simulink model "simulink_model_undamped"  (R2022b)
settings: Solver=ode5  StartTime=0.0  StopTime=10.0  RelTol=1e-3
settings Model: Creator=Cole  LastModifiedBy=Cole
settings DataIOCC: ReturnWorkspaceOutputs=off

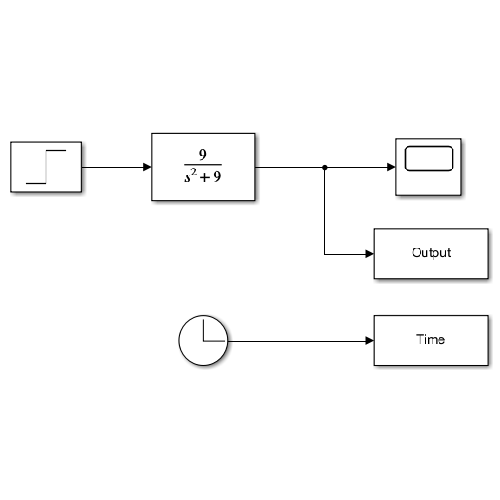
[thumbnail: Simulink's stored preview of the top-level diagram]
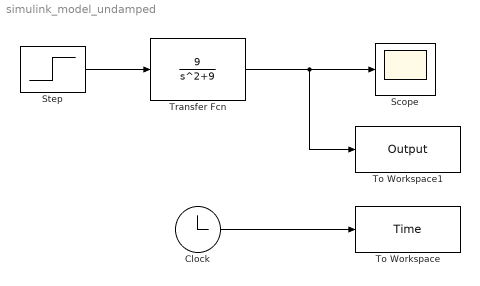
== system simulink_model_undamped ==
  Clock : Clock
  Scope : Scope
  Step : Step  Time=0  SampleTime=0
  To Workspace : ToWorkspace  VariableName=Time  SaveFormat=Timeseries  SampleTime=-1
  To Workspace1 : ToWorkspace  VariableName=Output  SaveFormat=Timeseries  SampleTime=-1
  Transfer Fcn : TransferFcn  Numerator=[9]  Denominator=[1 0 9]
  wires:
  Step/1 -> Transfer Fcn/1
  Transfer Fcn/1 -> Scope/1, To Workspace1/1
  Clock/1 -> To Workspace/1
